simulink model "acc"  (R2021b)
settings: Solver=FixedStepAuto  StartTime=0.0  StopTime=206  FixedStep=0.0005  RelTol=1e-3
values from neighbouring files (symbols this model uses):
  Leftdis_PV_switch = 2    [acc_plot_backup.m]
  s_path = [0 1.10508939428 2.2141958029 3.32141571172 4.42705301151 5.53154548532 6.63517443471 7.73808041313 8.84055018688 9.94289959674 11.0453539299 12.1480581097 ... (1001 elements, 1001x1)]    [200_100radius.mat]    (also in LV_Clothoid_S_Turn_path.mat = [0 0.966832089581 1.93621320584 2.90214024471 3.86476766313 ; NEDC_path.mat = [0 0.414605943146 0.832514087334 1.25401518562 1.68216660344; Straight_East_into_curve.mat = [0 1.65770560069 3.32192925577 4.98420060507 6.64484613518 8; acc_plot_backup.m = Station_HV_m)
  X_path = [0 1.10508939428 2.2141958029 3.32141571172 4.42705301151 5.53154548532 6.63517443471 7.73808041313 8.84055018688 9.94289959674 11.0453539299 12.1480581097 ... (1001 elements, 1001x1)]    [200_100radius.mat]    (also in LV_Clothoid_S_Turn_path.mat = [-10 -9.03316791042 -8.06378679416 -7.09785975529 -6.1352323; NEDC_path.mat = [0 0.414605943146 0.832514087334 1.25401518562 1.68216660344; Straight_East_into_curve.mat = [0 1.65770560069 3.32192925577 4.98420060507 6.64484613518 8; acc_plot_backup.m = X_HV_m)
  Y_path = [0 -1.70364610795e-18 -7.41532896709e-18 1.46822109542e-17 4.74557362791e-17 6.12980216762e-17 9.25043977736e-17 1.24088240159e-16 1.5099156923e-16 1.7058517853e-16 1.90629227614e-16 2.09673434424e-16 ... (1001 elements, 1001x1)]    [200_100radius.mat]    (also in LV_Clothoid_S_Turn_path.mat = [0 -8.46153035536e-19 5.07382551045e-18 2.07356032218e-17 3.; NEDC_path.mat = [0 -3.50680326162e-18 -2.14111304971e-18 3.38197671014e-18 3; Straight_East_into_curve.mat = [0 1.29197709199e-18 2.81882429322e-18 3.49020462564e-17 6.7; acc_plot_backup.m = Y_HV_m)
undefined symbols (not defined in the file or in its folder): C_TICK_TIME_S, ENUM_ACCSTATE_DISABLED, ENUM_ACCSTATE_OFF, ENUM_ACCSTATE_STANDBY, FALSE, KVDI_ACCLongPressTime_ms, KVDI_ACCMaxActSpeed_kph, KVDI_ACCSetSpdIntial_kph, KVDI_ACCSpdLargeChange_kph, KVDI_LongPressConTime_ms, ONE_FLOAT, ONE_INT, R, Rw, T, TRUE, ZERO_FLOAT, ZERO_INT
libraries: simulink x16, dspstat3 x4, simulink_extras x2, Solver_SF x1
(part 2 of 4)

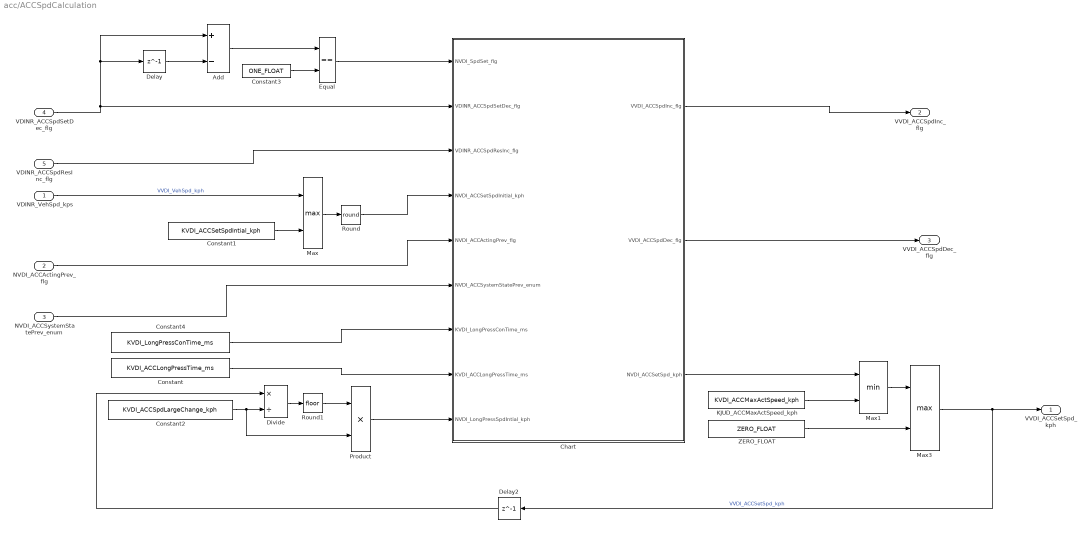
== system acc/ACCSpdCalculation ==
  VDINR_VehSpd_kps : Inport
  NVDI_ACCActingPrev_flg : Inport  Port=2
  NVDI_ACCSystemStatePrev_enum : Inport  Port=3
  VDINR_ACCSpdSetDec_flg : Inport  Port=4
  VDINR_ACCSpdResInc_flg : Inport  Port=5
  Add : Sum  Inputs=+-
  Chart : Stateflow chart  TreatAsAtomicUnit=on
      settings: PortSchema="{\"entries\":[{\"content\":{\"sides\":[{\"content\":{\"connectorIds\":[\"In1\",\"In2\",\"In3\",\"In4\",\"In5\",\"In6\",\"In9\",\"In7\",\"In8\"]},\"type\":\"ConnectorPlacement.EquallySpacedRectSide\",\"uuid\":\"b1b09059-7c6b-4f2a-a509-9d89abb69bff\"},{\"content\":{\"connectorIds\":[\"Out2\",\"Out3\",\"Out1\"],\"side\":\"RIGHT\"},\"type\":\"ConnectorPlacement.EquallySpacedRectSide\",\"uuid\":\"426eb2b7-8f84-437e-9ce1-b8172d5a5373\"},{\"content\":{\"connectorIds\":[],\"side\":\"TOP\"},\"type\":\"ConnectorPlacement.EquallySpacedRectSide\",\"uuid\":\"808310a0-6f78-4728-b2e8-69880cb1a9d0\"}]},\"type\":\"ConnectorPlacement.EquallySpacedConnector\",\"uuid\":\"50fcbb31-1c9a-4815-926e-b0772552613f\"}],\"packageUris\":[\"http://schema.mathworks.com/mf0/Connector/R2020b\"],\"version\":\"1.0\"}"
  Constant : Constant  Value=KVDI_ACCLongPressTime_ms
  Constant1 : Constant  Value=KVDI_ACCSetSpdIntial_kph
  Constant2 : Constant  Value=KVDI_ACCSpdLargeChange_kph
  Constant3 : Constant  Value=ONE_FLOAT
  Constant4 : Constant  Value=KVDI_LongPressConTime_ms
  Delay : Delay  DelayLength=1
  Delay2 : Delay  DelayLength=1
  Divide : Product  Inputs=*/
  Equal : RelationalOperator  Operator===  OutDataTypeStr=boolean  RndMeth=Simplest
  KJUD_ACCMaxActSpeed_kph : Constant  Value=KVDI_ACCMaxActSpeed_kph
  Max : MinMax  Function=max  Inputs=2
  Max1 : MinMax  Inputs=2
  Max3 : MinMax  Function=max  Inputs=2
  Product : Product
  Round : Rounding  Operator=round
  Round1 : Rounding
  ZERO_FLOAT : Constant  Value=ZERO_FLOAT
  VVDI_ACCSetSpd_kph : Outport
  VVDI_ACCSpdInc_flg : Outport  Port=2
  VVDI_ACCSpdDec_flg : Outport  Port=3
  wires:
  Constant4/1 -> Chart/9(KVDI_LongPressConTime_ms)
  Chart/2(VVDI_ACCSpdInc_flg) -> VVDI_ACCSpdInc_flg/1
  Chart/3(VVDI_ACCSpdDec_flg) -> VVDI_ACCSpdDec_flg/1
  Max1/1 -> Max3/1
  KJUD_ACCMaxActSpeed_kph/1 -> Max1/2
  VDINR_ACCSpdSetDec_flg/1 -> Chart/2(VDINR_ACCSpdSetDec_flg), Delay/1, Add/1
  Constant3/1 -> Equal/2
  Delay/1 -> Add/2
  Add/1 -> Equal/1
  Equal/1 -> Chart/1(NVDI_SpdSet_flg)
  ZERO_FLOAT/1 -> Max3/2
  Chart/1(NVDI_ACCSetSpd_kph) -> Max1/1
  Product/1 -> Chart/8(NVDI_LongPressSpdIntial_kph)
  Divide/1 -> Round1/1
  Round1/1 -> Product/1
  Constant2/1 -> Divide/2, Product/2
  Delay2/1 -> Divide/1
  Round/1 -> Chart/4(NVDI_ACCSetSpdInitial_kph)
  VDINR_VehSpd_kps/1 -> Max/1  "VVDI_VehSpd_kph"
  Constant1/1 -> Max/2
  Max/1 -> Round/1
  NVDI_ACCSystemStatePrev_enum/1 -> Chart/6(NVDI_ACCSystemStatePrev_enum)
  NVDI_ACCActingPrev_flg/1 -> Chart/5(NVDI_ACCActingPrev_flg)
  Max3/1 -> VVDI_ACCSetSpd_kph/1, Delay2/1  "VVDI_ACCSetSpd_kph"
  VDINR_ACCSpdResInc_flg/1 -> Chart/3(VDINR_ACCSpdResInc_flg)
  Constant/1 -> Chart/7(KVDI_ACCLongPressTime_ms)

== system acc/ACC_Mode_Selector ==
  ACCSetSpeed_mps : Inport
  VACCTargetVehNotAssigned_flg : Inport  Port=2
  RR : Inport  Port=3
  Vx_HV_mps : Inport  Port=4
  RV : Inport  Port=5
  Add : Sum
  Add13 : Sum  Inputs=+-
  Constant36 : Constant  Value=-0.5
  Logical Operator : Logic  Operator=OR  Inputs=3  AllPortsSameDT=off  OutDataTypeStr=boolean
  Logical Operator3 : Logic  AllPortsSameDT=off  OutDataTypeStr=boolean
  Relational Operator : RelationalOperator  Operator=<  OutDataTypeStr=boolean  RndMeth=Simplest
  Relational Operator1 : RelationalOperator  Operator=<  OutDataTypeStr=boolean  RndMeth=Simplest
  Relational Operator4 : RelationalOperator  Operator=<  OutDataTypeStr=boolean  RndMeth=Simplest
  TH_ref : Gain  Gain=1.5
  TH_ref4 : Gain  Gain=1.5
  dist_safe1 : Bias  Bias=-2
  Out1 : Outport
  wires:
  Logical Operator/1 -> Out1/1
  [Vx_PV_mps] -> Relational Operator/2
  VACCTargetVehNotAssigned_flg/1 -> Logical Operator/1
  Relational Operator/1 -> Logical Operator/2  "set_spd_compare"
  ACCSetSpeed_mps/1 -> [ACCSetSpeed_mps], Relational Operator/1
  Add/1 -> [Vx_PV_mps]
  Vx_HV_mps/1 -> [Vx_HV_mps], Add/2
  RV/1 -> Add/1
  dist_safe1/1 -> Add13/2, Relational Operator4/2  "act"
  TH_ref4/1 -> Relational Operator4/1  "des"
  Relational Operator1/1 -> Logical Operator3/1
  Constant36/1 -> Relational Operator1/2
  Add13/1 -> Relational Operator1/1
  Logical Operator3/1 -> Logical Operator/3  "dist_compare"
  RR/1 -> dist_safe1/1
  TH_ref/1 -> Add13/1  "des"
  [ACCSetSpeed_mps] -> TH_ref4/1
  [Vx_HV_mps] -> TH_ref/1
  Relational Operator4/1 -> Logical Operator3/2

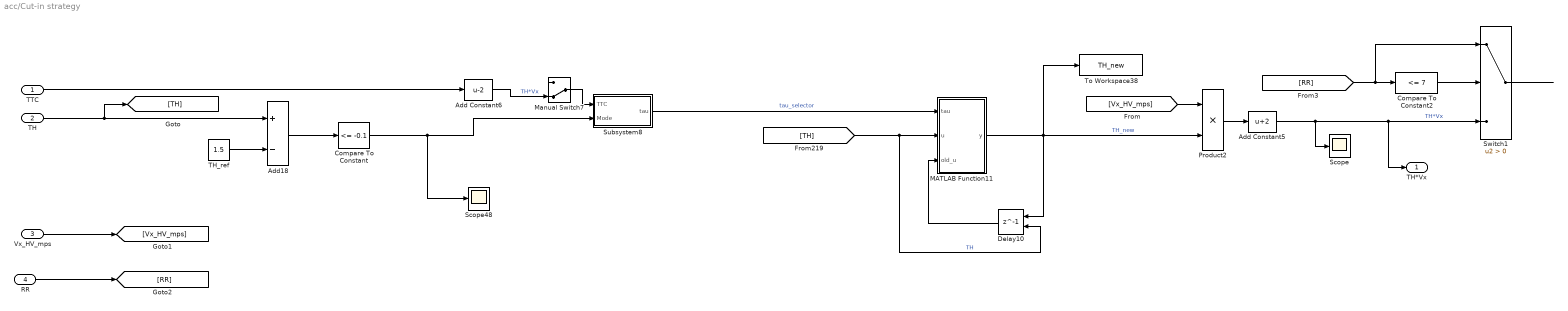
== system acc/Cut-in strategy ==
  TTC : Inport
  TH : Inport  Port=2
  Vx_HV_mps : Inport  Port=3
  RR : Inport  Port=4
  Add Constant5 : Bias  Bias=2
  Add Constant6 : Bias  Bias=-2
  Add18 : Sum  Inputs=+-
  Compare To Constant : simulink/Logic and Bit Operations/Compare To Constant  relop=<=  const=-0.1  OutDataTypeStr=boolean
  Compare To Constant2 : simulink/Logic and Bit Operations/Compare To Constant  relop=<=  const=7  OutDataTypeStr=boolean
  Delay10 : Delay  DelayLength=1  InitialConditionSource=Input port  SampleTime=0.1
      settings: InputPortMap=u0,p4
  MATLAB Function11 : MATLAB Function  TreatAsAtomicUnit=on
  Manual Switch7 : ManualSwitch  CurrentSetting=0
  Product2 : Product
  Scope : Scope
  Scope48 : Scope
  Subsystem8 : Subsystem
  Switch1 : Switch  Criteria=u2 > Threshold
  TH_ref : Constant  Value=1.5
  To Workspace38 : ToWorkspace  VariableName=TH_new  SampleTime=-1
  TH*Vx : Outport
  wires:
  [TH] -> Delay10/2, MATLAB Function11/2(u)  "TH"
  TH/1 -> Add18/1, [TH]
  Subsystem8/1(tau) -> MATLAB Function11/1(tau)  "tau_selector"
  Add18/1 -> Compare To Constant/1
  MATLAB Function11/1(y) -> Product2/2, To Workspace38/1, Delay10/1  "TH_new"
  Add Constant6/1 -> Manual Switch7/2  "TH*Vx"
  Delay10/1 -> MATLAB Function11/3(old_u)
  Product2/1 -> Add Constant5/1
  Manual Switch7/1 -> Subsystem8/1(TTC)
  TH_ref/1 -> Add18/2
  Compare To Constant/1 -> Scope48/1, Subsystem8/2(Mode)
  Add Constant5/1 -> Scope/1, TH*Vx/1, Switch1/3  "TH*Vx"
  [Vx_HV_mps] -> Product2/1
  TTC/1 -> Add Constant6/1
  Vx_HV_mps/1 -> [Vx_HV_mps]
  RR/1 -> [RR]
  [RR] -> Switch1/1, Compare To Constant2/1
  Compare To Constant2/1 -> Switch1/2
  Switch1/1 -> ?

== system acc/Latch ==
  set : Inport
  reset : Inport  Port=2
  Delay : Delay  DelayLength=1
  Logical Operator3 : Logic  AllPortsSameDT=off  OutDataTypeStr=boolean
  Logical Operator4 : Logic  Operator=NOT  AllPortsSameDT=off  OutDataTypeStr=boolean
  Switch : Switch  Criteria=u2 ~= 0
  Switch1 : Switch  Criteria=u2 ~= 0
  latched : Outport
  wires:
  Delay/1 -> Switch1/3
  Logical Operator4/1 -> Logical Operator3/2, Switch1/1
  Logical Operator3/1 -> Switch/2
  reset/1 -> Logical Operator4/1, Switch1/2
  Switch/1 -> Delay/1, latched/1
  set/1 -> Switch/1, Logical Operator3/1
  Switch1/1 -> Switch/3

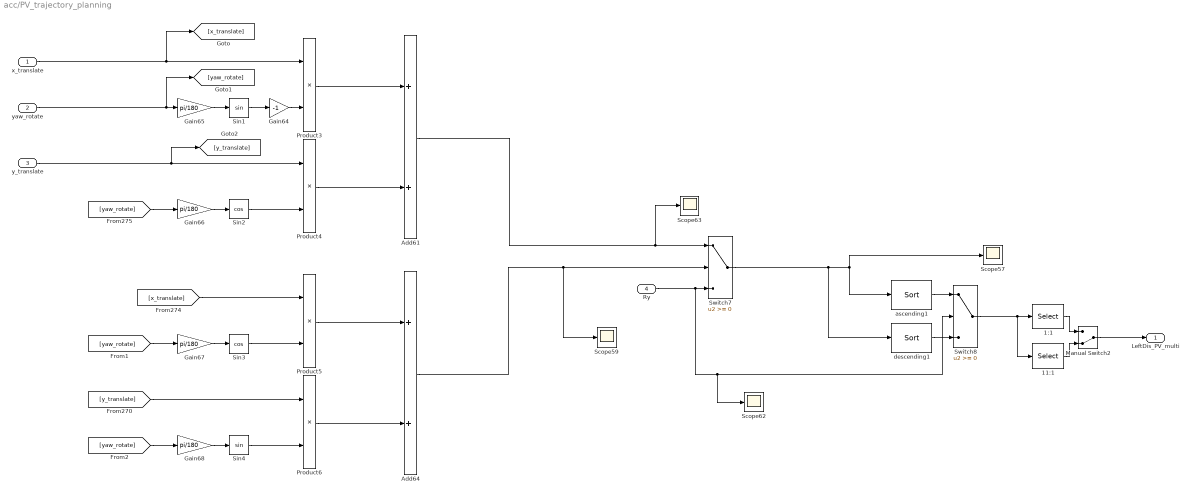
== system acc/PV_trajectory_planning ==
  x_translate : Inport
  yaw_rotate : Inport  Port=2
  y_translate : Inport  Port=3
  Ry : Inport  Port=4
  11:1 : Selector  InputPortWidth=20  IndexOptions=Index vector (dialog)  Indices=[11:20]  OutputSizes=1
  1:1 : Selector  InputPortWidth=20  IndexOptions=Index vector (dialog)  Indices=[1:10]  OutputSizes=1
  Add61 : Sum
  Add64 : Sum
  Gain64 : Gain  Gain=-1
  Gain{65..68} (4 alike) : Gain  Gain=pi/180
  Manual Switch2 : ManualSwitch  CurrentSetting=0
  Product{3..6} (4 alike) : Product
  Scope{57,59,62..63} (4 alike) : Scope
  Sin1 : Trigonometry
  Sin2 : Trigonometry  Operator=cos
  Sin3 : Trigonometry  Operator=cos
  Sin4 : Trigonometry
  Switch7 : Switch
  Switch8 : Switch
  ascending1 : dspstat3/Sort  otype=Value  dir=Ascending  sortAlg=Quick sort  roundingMode=Floor  overflowMode=off  accumDataTypeStr=Inherit: Same as product output  accumLastDataTypeStr=Inherit: Same as product output
      settings: SourceProductBaseCode=DS
  descending1 : dspstat3/Sort  otype=Value  dir=Descending  sortAlg=Quick sort  roundingMode=Floor  overflowMode=off  accumDataTypeStr=Inherit: Same as product output  accumLastDataTypeStr=Inherit: Same as product output
      settings: SourceProductBaseCode=DS
  LeftDis_PV_multi : Outport
  wires:
  Add64/1 -> Scope59/1, Switch7/2
  Product5/1 -> Add64/1
  Gain68/1 -> Sin4/1
  Sin1/1 -> Gain64/1
  Gain64/1 -> Product3/2
  descending1/1 -> Switch8/3
  Ry/1 -> Scope62/1, Switch8/2, Switch7/3
  Sin4/1 -> Product6/2
  Gain67/1 -> Sin3/1
  Switch8/1 -> 11:1/1, 1:1/1
  [yaw_rotate] -> Gain68/1
  Sin3/1 -> Product5/2
  Product6/1 -> Add64/2
  Switch7/1 -> Scope57/1, ascending1/1, descending1/1
  Sin2/1 -> Product4/2
  Gain66/1 -> Sin2/1
  y_translate/1 -> [y_translate], Product4/1
  Gain65/1 -> Sin1/1
  [x_translate] -> Product5/1
  ascending1/1 -> Switch8/1
  1:1/1 -> Manual Switch2/1
  Product4/1 -> Add61/2
  11:1/1 -> Manual Switch2/2
  Add61/1 -> Scope63/1, Switch7/1
  Product3/1 -> Add61/1
  Manual Switch2/1 -> LeftDis_PV_multi/1
  x_translate/1 -> Product3/1, [x_translate]
  [y_translate] -> Product6/1
  [yaw_rotate] -> Gain67/1
  yaw_rotate/1 -> [yaw_rotate], Gain65/1
  [yaw_rotate] -> Gain66/1

== system acc/R selector ==
  In1 : Inport
  vx : Inport  Port=2
  1-D Lookup Table2 : Lookup_n-D  NumberOfTableDimensions=1  BreakpointsForDimension1=[0 15 28 40]/3.6  Table=[31 31 35 35]  InternalRulePriority=Speed  RndMeth=Simplest  InputSameDT=on
  Constant1 : Constant  Value=35
  Constant19 : Constant
  Constant2 : Constant  Value=20
  Constant66 : Constant  Value=0.5
  Switch12 : Switch  Criteria=u2 > Threshold
  Out1 : Outport
  wires:
  Constant66/1 -> Switch12/1
  1-D Lookup Table2/1 -> Switch12/3
  In1/1 -> Switch12/2
  Switch12/1 -> Out1/1
  vx/1 -> 1-D Lookup Table2/1

== system acc/R selector1 ==
  In1 : Inport
  vx : Inport  Port=2
  1-D Lookup Table2 : Lookup_n-D  NumberOfTableDimensions=1  BreakpointsForDimension1=[0 15 28 40]/3.6  Table=[31 31 35 35]  InternalRulePriority=Speed  RndMeth=Simplest  InputSameDT=on
  Constant1 : Constant  Value=35
  Constant19 : Constant
  Constant2 : Constant  Value=7
  Constant66 : Constant  Value=0.5
  Switch12 : Switch  Criteria=u2 > Threshold
  Out1 : Outport
  wires:
  Switch12/1 -> Out1/1
  In1/1 -> Switch12/2
  Constant2/1 -> Switch12/3
  Constant66/1 -> Switch12/1

== system acc/Smooth Switch ==
  Spd_acc_cmd : Inport
  Mode : Inport  Port=2
  TH_acc_cmd : Inport  Port=3
  TTC : Inport  Port=4
  Add12 : Sum
  Add9 : Sum  Inputs=+-
  Constant49 : Constant
  Data Type Conversion : DataTypeConversion  OutDataTypeStr=double
  Delay : Delay  DelayLength=1  InitialConditionSource=Input port  SampleTime=0.1
      settings: InputPortMap=u0,p4
  MATLAB Function : MATLAB Function  TreatAsAtomicUnit=on
  Product1 : Product
  Product2 : Product
  Scope : Scope
  Subsystem : Subsystem
  ax_cmd : Outport
  wires:
  Product2/1 -> Add12/1
  Spd_acc_cmd/1 -> Product2/1
  MATLAB Function/1(y) -> Delay/1, Scope/1, Add9/2, Product2/2
  Data Type Conversion/1 -> Delay/2, MATLAB Function/2(u)
  Constant49/1 -> Add9/1
  Product1/1 -> Add12/2
  TH_acc_cmd/1 -> Product1/2
  Add9/1 -> Product1/1
  Add12/1 -> ax_cmd/1
  Mode/1 -> Subsystem/2(Mode), Data Type Conversion/1
  Delay/1 -> MATLAB Function/3(old_u)
  Subsystem/1(tau) -> MATLAB Function/1(tau)  "tau_selector"
  TTC/1 -> Subsystem/1(TTC)

== system acc/Smooth Switch1 ==
  Dynamic_cmd : Inport
  Mode : Inport  Port=2
  Kinematic_cmd : Inport  Port=3
  Add12 : Sum
  Add9 : Sum  Inputs=+-
  Constant49 : Constant
  Data Type Conversion : DataTypeConversion  OutDataTypeStr=double
  Product1 : Product
  Product2 : Product
  Transfer Fcn5 : TransferFcn  Denominator=[0.5 1]
  ax_cmd : Outport
  wires:
  Mode/1 -> Data Type Conversion/1
  Add12/1 -> ax_cmd/1
  Add9/1 -> Product1/1
  Kinematic_cmd/1 -> Product1/2
  Product1/1 -> Add12/2
  Constant49/1 -> Add9/1
  Data Type Conversion/1 -> Transfer Fcn5/1
  Transfer Fcn5/1 -> Product2/2, Add9/2
  Dynamic_cmd/1 -> Product2/1
  Product2/1 -> Add12/1

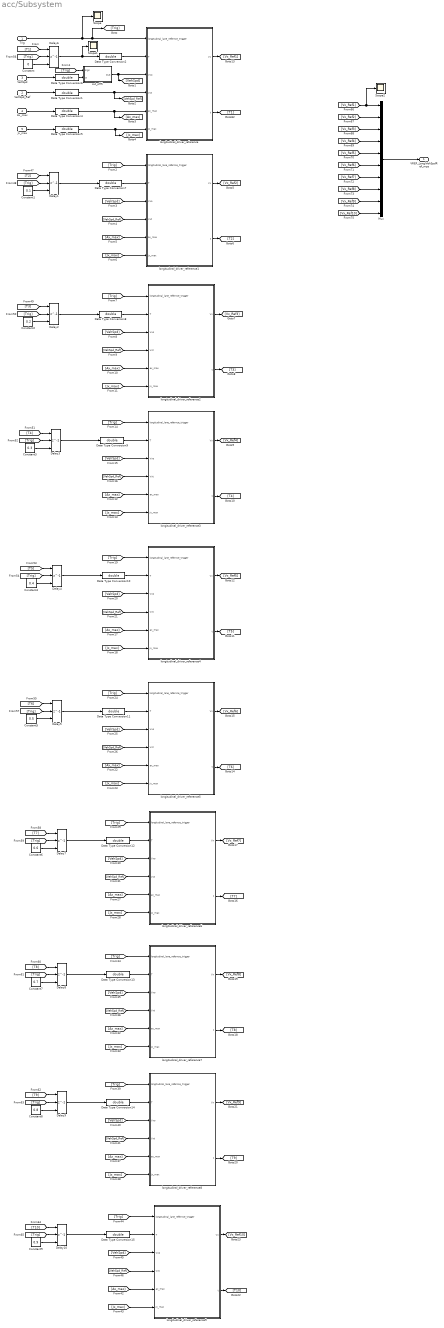
== system acc/Subsystem ==
  "Trig " : Inport
  VehSpd_Ref : Inport  Port=2
  VehSpd : Inport  Port=3
  Ax_max : Inport  Port=4
  Jx_max : Inport  Port=5
  Constant : Constant  Value=0
  Constant1 : Constant  Value=0.1
  Constant2 : Constant  Value=0.2
  Constant3 : Constant  Value=0.3
  Constant4 : Constant  Value=0.4
  Constant5 : Constant  Value=0.5
  Constant6 : Constant  Value=0.6
  Constant7 : Constant  Value=0.7
  Constant8 : Constant  Value=0.8
  Constant9 : Constant  Value=0.9
  Data Type Conversion{1..2,4..15} (14 alike) : DataTypeConversion  OutDataTypeStr=double
  Delay{1..10} (10 alike) : Delay  DelayLength=1  InitialConditionSource=Input port  ExternalReset=Rising
      settings: InputPortMap=u0,r5,p4
  Mux : Mux  Inputs=10
  Scope : Scope
  Scope1 : Scope
  Scope2 : Scope
  cut_off5 : Subsystem
  longitudinal_driver_reference : MATLAB Function  TreatAsAtomicUnit=on
  longitudinal_driver_reference1 : MATLAB Function  TreatAsAtomicUnit=on
  longitudinal_driver_reference2 : MATLAB Function  TreatAsAtomicUnit=on
  longitudinal_driver_reference3 : MATLAB Function  TreatAsAtomicUnit=on
  longitudinal_driver_reference4 : MATLAB Function  TreatAsAtomicUnit=on
  longitudinal_driver_reference5 : MATLAB Function  TreatAsAtomicUnit=on
  longitudinal_driver_reference6 : MATLAB Function  TreatAsAtomicUnit=on
  longitudinal_driver_reference7 : MATLAB Function  TreatAsAtomicUnit=on
  longitudinal_driver_reference8 : MATLAB Function  TreatAsAtomicUnit=on
  longitudinal_driver_reference9 : MATLAB Function  TreatAsAtomicUnit=on
  "VREF_LongiVehSpdRef_mps " : Outport
  wires:
  longitudinal_driver_reference/1(Vx) -> [Vx_Ref1]
  Mux/1 -> "VREF_LongiVehSpdRef_mps "/1
  Constant/1 -> Delay6/3
  [T1] -> Delay6/1
  Ax_max/1 -> Data Type Conversion4/1
  Jx_max/1 -> Data Type Conversion5/1
  VehSpd_Ref/1 -> Data Type Conversion1/1
  longitudinal_driver_reference/2(t) -> [T1]
  Delay6/1 -> Scope1/1, Data Type Conversion2/1
  [Trig] -> Delay6/2
  "Trig "/1 -> Scope/1, [Trig], longitudinal_driver_reference/1(longitudinal_lane_refernce_trigger)
  Data Type Conversion2/1 -> longitudinal_driver_reference/2(T)
  VehSpd/1 -> Data Type Conversion6/1
  Data Type Conversion1/1 -> [VehSpd_Ref], longitudinal_driver_reference/4(Vxt)
  cut_off5/1(Out) -> [VehSpd], longitudinal_driver_reference/3(Vxo)
  Data Type Conversion6/1 -> cut_off5/2(in)
  [Trig] -> cut_off5/1(sign)
  Data Type Conversion5/1 -> [Jx_max], longitudinal_driver_reference/6(jx_max)
  Data Type Conversion4/1 -> [Ax_max], longitudinal_driver_reference/5(ax_max)
  [Trig] -> longitudinal_driver_reference1/1(longitudinal_lane_refernce_trigger)
  [VehSpd] -> longitudinal_driver_reference1/3(Vxo)
  [VehSpd_Ref] -> longitudinal_driver_reference1/4(Vxt)
  [Ax_max] -> longitudinal_driver_reference1/5(ax_max)
  [Jx_max] -> longitudinal_driver_reference1/6(jx_max)
  [Jx_max] -> longitudinal_driver_reference2/6(jx_max)
  [Ax_max] -> longitudinal_driver_reference2/5(ax_max)
  [VehSpd_Ref] -> longitudinal_driver_reference2/4(Vxt)
  [VehSpd] -> longitudinal_driver_reference2/3(Vxo)
  [Trig] -> longitudinal_driver_reference2/1(longitudinal_lane_refernce_trigger)
  [Trig] -> longitudinal_driver_reference3/1(longitudinal_lane_refernce_trigger)
  [VehSpd] -> longitudinal_driver_reference3/3(Vxo)
  [VehSpd_Ref] -> longitudinal_driver_reference3/4(Vxt)
  [Ax_max] -> longitudinal_driver_reference3/5(ax_max)
  [Jx_max] -> longitudinal_driver_reference3/6(jx_max)
  [Jx_max] -> longitudinal_driver_reference4/6(jx_max)
  [Ax_max] -> longitudinal_driver_reference4/5(ax_max)
  [VehSpd_Ref] -> longitudinal_driver_reference4/4(Vxt)
  [VehSpd] -> longitudinal_driver_reference4/3(Vxo)
  [Trig] -> longitudinal_driver_reference4/1(longitudinal_lane_refernce_trigger)
  [Trig] -> longitudinal_driver_reference5/1(longitudinal_lane_refernce_trigger)
  [VehSpd] -> longitudinal_driver_reference5/3(Vxo)
  [VehSpd_Ref] -> longitudinal_driver_reference5/4(Vxt)
  [Ax_max] -> longitudinal_driver_reference5/5(ax_max)
  [Jx_max] -> longitudinal_driver_reference5/6(jx_max)
  [Jx_max] -> longitudinal_driver_reference6/6(jx_max)
  [Ax_max] -> longitudinal_driver_reference6/5(ax_max)
  [VehSpd_Ref] -> longitudinal_driver_reference6/4(Vxt)
  [VehSpd] -> longitudinal_driver_reference6/3(Vxo)
  [Trig] -> longitudinal_driver_reference6/1(longitudinal_lane_refernce_trigger)
  [Trig] -> longitudinal_driver_reference7/1(longitudinal_lane_refernce_trigger)
  [VehSpd] -> longitudinal_driver_reference7/3(Vxo)
  [VehSpd_Ref] -> longitudinal_driver_reference7/4(Vxt)
  [Ax_max] -> longitudinal_driver_reference7/5(ax_max)
  [Jx_max] -> longitudinal_driver_reference7/6(jx_max)
  [Jx_max] -> longitudinal_driver_reference8/6(jx_max)
  [Ax_max] -> longitudinal_driver_reference8/5(ax_max)
  [VehSpd_Ref] -> longitudinal_driver_reference8/4(Vxt)
  [VehSpd] -> longitudinal_driver_reference8/3(Vxo)
  [Trig] -> longitudinal_driver_reference8/1(longitudinal_lane_refernce_trigger)
  [Trig] -> longitudinal_driver_reference9/1(longitudinal_lane_refernce_trigger)
  [VehSpd] -> longitudinal_driver_reference9/3(Vxo)
  [VehSpd_Ref] -> longitudinal_driver_reference9/4(Vxt)
  [Ax_max] -> longitudinal_driver_reference9/5(ax_max)
  [Jx_max] -> longitudinal_driver_reference9/6(jx_max)
  longitudinal_driver_reference1/1(Vx) -> [Vx_Ref2]
  longitudinal_driver_reference1/2(t) -> [T2]
  [Trig] -> Delay1/2
  Delay1/1 -> Data Type Conversion7/1
  [T2] -> Delay1/1
  Data Type Conversion7/1 -> longitudinal_driver_reference1/2(T)
  Constant1/1 -> Delay1/3
  Constant2/1 -> Delay2/3
  Data Type Conversion8/1 -> longitudinal_driver_reference2/2(T)
  [T3] -> Delay2/1
  Delay2/1 -> Data Type Conversion8/1
  [Trig] -> Delay2/2
  longitudinal_driver_reference2/2(t) -> [T3]
  longitudinal_driver_reference2/1(Vx) -> [Vx_Ref3]
  [Trig] -> Delay3/2
  Delay3/1 -> Data Type Conversion9/1
  [T4] -> Delay3/1
  Data Type Conversion9/1 -> longitudinal_driver_reference3/2(T)
  Constant3/1 -> Delay3/3
  longitudinal_driver_reference3/1(Vx) -> [Vx_Ref4]
  longitudinal_driver_reference3/2(t) -> [T4]
  Constant4/1 -> Delay4/3
  Data Type Conversion10/1 -> longitudinal_driver_reference4/2(T)
  [T5] -> Delay4/1
  Delay4/1 -> Data Type Conversion10/1
  [Trig] -> Delay4/2
  longitudinal_driver_reference4/2(t) -> [T5]
  longitudinal_driver_reference4/1(Vx) -> [Vx_Ref5]
  longitudinal_driver_reference5/1(Vx) -> [Vx_Ref6]
  longitudinal_driver_reference5/2(t) -> [T6]
  [Trig] -> Delay5/2
  Delay5/1 -> Data Type Conversion11/1
  [T6] -> Delay5/1
  Constant5/1 -> Delay5/3
  Data Type Conversion11/1 -> longitudinal_driver_reference5/2(T)
  longitudinal_driver_reference6/2(t) -> [T7]
  longitudinal_driver_reference6/1(Vx) -> [Vx_Ref7]
  Constant6/1 -> Delay7/3
  [T7] -> Delay7/1
  Delay7/1 -> Data Type Conversion12/1
  [Trig] -> Delay7/2
  Data Type Conversion12/1 -> longitudinal_driver_reference6/2(T)
  [Trig] -> Delay8/2
  Delay8/1 -> Data Type Conversion13/1
  [T8] -> Delay8/1
  Constant7/1 -> Delay8/3
  Data Type Conversion13/1 -> longitudinal_driver_reference7/2(T)
  longitudinal_driver_reference7/1(Vx) -> [Vx_Ref8]
  longitudinal_driver_reference7/2(t) -> [T8]
  longitudinal_driver_reference8/2(t) -> [T9]
  longitudinal_driver_reference8/1(Vx) -> [Vx_Ref9]
  Data Type Conversion14/1 -> longitudinal_driver_reference8/2(T)
  Constant8/1 -> Delay9/3
  [T9] -> Delay9/1
  Delay9/1 -> Data Type Conversion14/1
  [Trig] -> Delay9/2
  longitudinal_driver_reference9/1(Vx) -> [Vx_Ref10]
  longitudinal_driver_reference9/2(t) -> [T10]
  [Trig] -> Delay10/2
  Delay10/1 -> Data Type Conversion15/1
  [T10] -> Delay10/1
  Constant9/1 -> Delay10/3
  Data Type Conversion15/1 -> longitudinal_driver_reference9/2(T)
  [Vx_Ref1] -> Scope2/1, Mux/1
  [Vx_Ref2] -> Mux/2
  [Vx_Ref3] -> Mux/3
  [Vx_Ref4] -> Mux/4
  [Vx_Ref5] -> Mux/5
  [Vx_Ref6] -> Mux/6
  [Vx_Ref7] -> Mux/7
  [Vx_Ref8] -> Mux/8
  [Vx_Ref9] -> Mux/9
  [Vx_Ref10] -> Mux/10

== system acc/Subsystem1 ==
  In1 : Inport
  Constant117 : Constant  Value=single(1)  OutDataTypeStr=single
  Relational Operator : RelationalOperator  OutDataTypeStr=boolean  RndMeth=Simplest
  Saturation5 : Saturate  UpperLimit=inf  LowerLimit=40/3.6
  Switch7 : Switch  Criteria=u2 ~= 0
  Out1 : Outport
  wires:
  Relational Operator/1 -> Switch7/2
  In1/1 -> Relational Operator/1, Switch7/1
  Constant117/1 -> Relational Operator/2, Switch7/3
  Switch7/1 -> Out1/1

== system acc/Subsystem16 ==
  C0 : Inport
  C1 : Inport  Port=2
  "C2 " : Inport  Port=3
  C3 : Inport  Port=4
  PrediDis : Inport  Port=5
  Add30 : Sum  Inputs=++++
  Fcn : Fcn  Expr=(u)^3
  Product : Product
  Product1 : Product
  Product2 : Product
  Square : Math  Operator=square  SignedPower=on  RndMeth=Zero  SaturateOnIntegerOverflow=on
  LeftDis : Outport  VectorParamsAs1DForOutWhenUnconnected=off
  wires:
  PrediDis/1 -> [PrediDis]
  [PrediDis] -> Square/1
  Product/1 -> Add30/2
  Product1/1 -> Add30/3
  "C2 "/1 -> Product1/1
  [PrediDis] -> Product/2
  [PrediDis] -> Fcn/1
  Fcn/1 -> Product2/2
  Square/1 -> Product1/2
  C0/1 -> Add30/1
  Product2/1 -> Add30/4
  C1/1 -> Product/1
  Add30/1 -> LeftDis/1
  C3/1 -> Product2/1

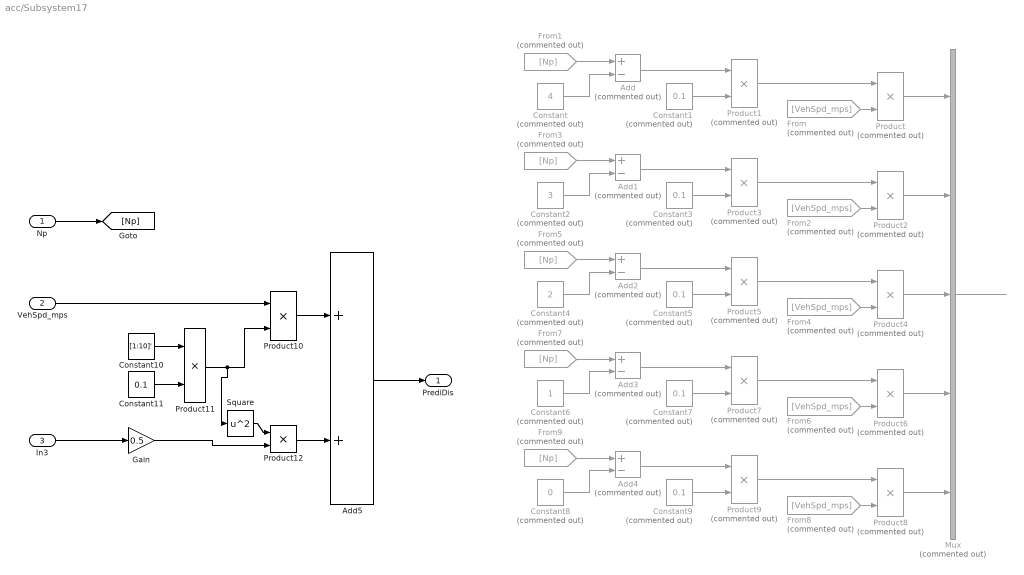
== system acc/Subsystem17 ==
  Np : Inport
  VehSpd_mps : Inport  Port=2
  In3 : Inport  Port=3
  Add{,1..4} (5 alike) : Sum  Commented=on  Inputs=+-
  Add5 : Sum
  Constant : Constant  Commented=on  Value=4
  Constant{1,3,5,7,9} (5 alike) : Constant  Commented=on  Value=0.1
  Constant10 : Constant  Value=[1:10]'
  Constant11 : Constant  Value=0.1
  Constant2 : Constant  Commented=on  Value=3
  Constant4 : Constant  Commented=on  Value=2
  Constant6 : Constant  Commented=on
  Constant8 : Constant  Commented=on  Value=0
  From{,2,4,6,8} (5 alike) : From  Commented=on  GotoTag=VehSpd_mps
  From{1,3,5,7,9} (5 alike) : From  Commented=on  GotoTag=Np
  Gain : Gain  Gain=0.5
  Mux : Mux  Commented=on  Inputs=5
  Product{,1..9} (10 alike) : Product  Commented=on
  Product10 : Product
  Product11 : Product
  Product12 : Product
  Square : Math  Operator=square  SaturateOnIntegerOverflow=on
  PrediDis : Outport  VectorParamsAs1DForOutWhenUnconnected=off
  wires:
  Product8/1 -> Mux/5
  Constant9/1 -> Product9/2
  Constant8/1 -> Add4/2
  From9/1 -> Add4/1
  Add4/1 -> Product9/1
  Product9/1 -> Product8/1
  From8/1 -> Product8/2
  From6/1 -> Product6/2
  Product7/1 -> Product6/1
  Add3/1 -> Product7/1
  From7/1 -> Add3/1
  Constant6/1 -> Add3/2
  Constant7/1 -> Product7/2
  Product6/1 -> Mux/4
  Product4/1 -> Mux/3
  Constant5/1 -> Product5/2
  Constant4/1 -> Add2/2
  From5/1 -> Add2/1
  Add2/1 -> Product5/1
  Product5/1 -> Product4/1
  From4/1 -> Product4/2
  Product2/1 -> Mux/2
  From2/1 -> Product2/2
  Product3/1 -> Product2/1
  Add1/1 -> Product3/1
  From3/1 -> Add1/1
  Constant2/1 -> Add1/2
  Constant3/1 -> Product3/2
  Constant1/1 -> Product1/2
  Constant/1 -> Add/2
  From1/1 -> Add/1
  Add/1 -> Product1/1
  Product1/1 -> Product/1
  From/1 -> Product/2
  Product/1 -> Mux/1
  Np/1 -> [Np]
  Mux/1 -> ?
  Product10/1 -> Add5/1
  VehSpd_mps/1 -> Product10/1
  Product11/1 -> Product10/2, Square/1
  Constant10/1 -> Product11/1
  Constant11/1 -> Product11/2
  Add5/1 -> PrediDis/1
  In3/1 -> Gain/1
  Product12/1 -> Add5/2
  Square/1 -> Product12/1
  Gain/1 -> Product12/2

== system acc/Subsystem2 ==
  T_cmd : Inport
  Gain : Gain  Gain=-0.25
  Gain2 : Gain  Gain=1/250
  Gain3 : Gain  Gain=1/150
  Saturation1 : Saturate  UpperLimit=0  LowerLimit=-inf
  Smooth_Switch1 : Subsystem  Commented=on  mask{tau=0.3, IC=0, T=0.1}
      mask prompts: tau "Time constant"; T "Sample time"
      mask Display:
      | fprintf('Discrete first order \n\n')
      | fprintf(['tau=' num2str(tau) '    IC=' num2str(IC)])
  Transfer Fcn1 : TransferFcn  Denominator=[0.3 1]
  Transfer Fcn2 : TransferFcn  Denominator=[0.3 1]
  Pb_LF : Outport
  Pb_RF : Outport  Port=2
  Pb_RL : Outport  Port=3
  Pb_RR : Outport  Port=4
  wires:
  Transfer Fcn1/1 -> Pb_RR/1, Pb_RL/1
  Transfer Fcn2/1 -> Pb_RF/1, Pb_LF/1
  Gain3/1 -> Transfer Fcn1/1
  Gain2/1 -> Transfer Fcn2/1
  Gain/1 -> Gain2/1, Gain3/1
  Saturation1/1 -> Gain/1
  T_cmd/1 -> Saturation1/1

== system acc/Subsystem3 ==
  Jerk : Inport
  Vx : Inport  Port=2
  Constant1 : Constant  Value=0  OutDataTypeStr=single
  Constant117 : Constant  Value=0.5  OutDataTypeStr=single
  Relational Operator : RelationalOperator  OutDataTypeStr=boolean  RndMeth=Simplest
  Switch7 : Switch  Criteria=u2 ~= 0
  Out1 : Outport
  wires:
  Relational Operator/1 -> Switch7/2
  Vx/1 -> Relational Operator/1
  Constant117/1 -> Relational Operator/2
  Switch7/1 -> Out1/1
  Constant1/1 -> Switch7/3
  Jerk/1 -> Switch7/1

== system acc/Subsystem4 ==
  new_value : Inport
  Constant44 : Constant  Value=0.25
  Constant48 : Constant  Value=0.1
  Delay1 : Delay  DelayLength=1  SampleTime=0.1
  rolling_avg1 : Subsystem
  new_ave : Outport
  wires:
  Constant44/1 -> rolling_avg1/4(tc)
  new_value/1 -> rolling_avg1/1(new_value)
  Constant48/1 -> rolling_avg1/3(delta_t)  "T"
  Delay1/1 -> rolling_avg1/2(old_ave)
  rolling_avg1/1(new_ave) -> new_ave/1, Delay1/1

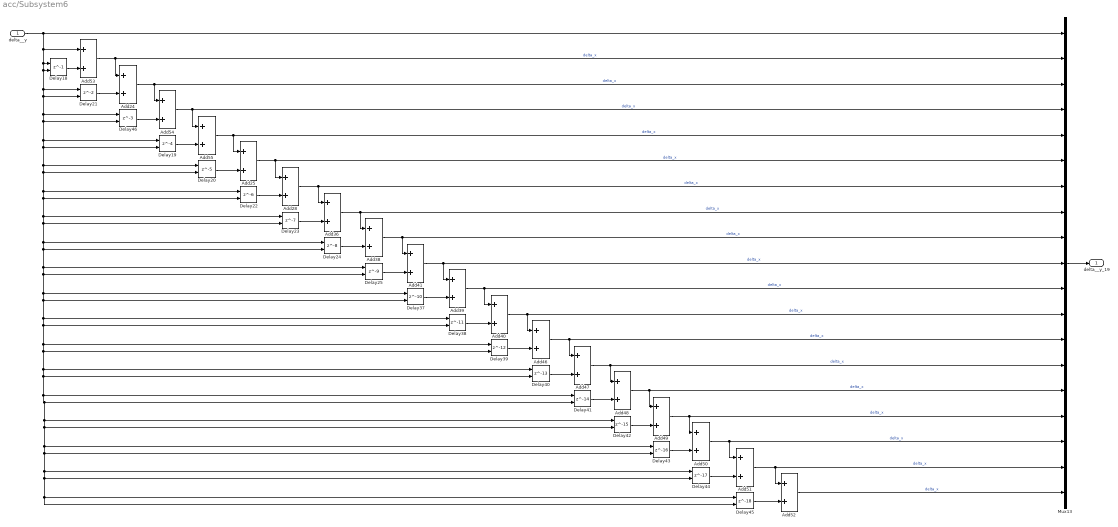
== system acc/Subsystem6 ==
  delta__y : Inport
  Add{24..25,28,36,38..41,46..55} (18 alike) : Sum
  Delay18 : Delay  DelayLength=1  InitialConditionSource=Input port
      settings: InputPortMap=u0,p4
  Delay19 : Delay  DelayLength=4  InitialConditionSource=Input port
      settings: InputPortMap=u0,p4
  Delay20 : Delay  DelayLength=5  InitialConditionSource=Input port
      settings: InputPortMap=u0,p4
  Delay21 : Delay  InitialConditionSource=Input port
      settings: InputPortMap=u0,p4
  Delay22 : Delay  DelayLength=6  InitialConditionSource=Input port
      settings: InputPortMap=u0,p4
  Delay23 : Delay  DelayLength=7  InitialConditionSource=Input port
      settings: InputPortMap=u0,p4
  Delay24 : Delay  DelayLength=8  InitialConditionSource=Input port
      settings: InputPortMap=u0,p4
  Delay25 : Delay  DelayLength=9  InitialConditionSource=Input port
      settings: InputPortMap=u0,p4
  Delay37 : Delay  DelayLength=10  InitialConditionSource=Input port
      settings: InputPortMap=u0,p4
  Delay38 : Delay  DelayLength=11  InitialConditionSource=Input port
      settings: InputPortMap=u0,p4
  Delay39 : Delay  DelayLength=12  InitialConditionSource=Input port
      settings: InputPortMap=u0,p4
  Delay40 : Delay  DelayLength=13  InitialConditionSource=Input port
      settings: InputPortMap=u0,p4
  Delay41 : Delay  DelayLength=14  InitialConditionSource=Input port
      settings: InputPortMap=u0,p4
  Delay42 : Delay  DelayLength=15  InitialConditionSource=Input port
      settings: InputPortMap=u0,p4
  Delay43 : Delay  DelayLength=16  InitialConditionSource=Input port
      settings: InputPortMap=u0,p4
  Delay44 : Delay  DelayLength=17  InitialConditionSource=Input port
      settings: InputPortMap=u0,p4
  Delay45 : Delay  DelayLength=18  InitialConditionSource=Input port
      settings: InputPortMap=u0,p4
  Delay46 : Delay  DelayLength=3  InitialConditionSource=Input port
      settings: InputPortMap=u0,p4
  Mux13 : Mux  Inputs=19
  delta__y_19 : Outport
  wires:
  Delay21/1 -> Add24/2
  delta__y/1 -> Mux13/1, Delay21/2, Delay46/1, Delay22/1, Delay25/2, Delay37/1, Delay39/2, Delay40/1, Delay41/1, Delay42/1, Delay42/2, Delay43/1, Delay44/1, Delay45/1, Delay45/2, Delay44/2, Delay43/2, Delay41/2, Delay40/2, Delay39/1, Delay38/2, Delay38/1, Delay37/2, Delay25/1, Delay24/2, Delay24/1, Delay23/2, Delay23/1, Delay22/2, Delay20/2, Delay20/1, Delay19/2, Delay19/1, Delay46/2, Delay21/1, Delay18/2, Delay18/1, Add53/1
  Delay22/1 -> Add28/2
  Add46/1 -> Mux13/13, Add47/1  "delta_x"
  Delay37/1 -> Add39/2
  Add39/1 -> Mux13/11, Add40/1  "delta_x"
  Delay38/1 -> Add40/2
  Add40/1 -> Mux13/12, Add46/1  "delta_x"
  Add38/1 -> Mux13/9, Add41/1  "delta_x"
  Add53/1 -> Mux13/2, Add24/1  "delta_x"
  Add55/1 -> Mux13/5, Add25/1  "delta_x"
  Add50/1 -> Add51/1, Mux13/17  "delta_x"
  Add47/1 -> Mux13/14, Add48/1  "delta_x"
  Delay39/1 -> Add46/2
  Delay40/1 -> Add47/2
  Mux13/1 -> delta__y_19/1
  Delay46/1 -> Add54/2
  Delay25/1 -> Add41/2
  Add52/1 -> Mux13/19  "delta_x"
  Add28/1 -> Mux13/7, Add36/1  "delta_x"
  Add36/1 -> Mux13/8, Add38/1  "delta_x"
  Delay23/1 -> Add36/2
  Delay20/1 -> Add25/2
  Delay42/1 -> Add49/2
  Delay44/1 -> Add51/2
  Delay18/1 -> Add53/2
  Add25/1 -> Mux13/6, Add28/1  "delta_x"
  Add41/1 -> Mux13/10, Add39/1  "delta_x"
  Add49/1 -> Add50/1, Mux13/16  "delta_x"
  Add51/1 -> Add52/1, Mux13/18  "delta_x"
  Delay19/1 -> Add55/2
  Add24/1 -> Mux13/3, Add54/1  "delta_x"
  Delay45/1 -> Add52/2
  Delay41/1 -> Add48/2
  Add54/1 -> Mux13/4, Add55/1  "delta_x"
  Delay24/1 -> Add38/2
  Delay43/1 -> Add50/2
  Add48/1 -> Mux13/15, Add49/1  "delta_x"

== system acc/V_rel Estimation ==
  cut_in_flg : Inport
  a_c : Inport  Port=2
  S_rel : Inport  Port=3
  initial_value : Inport  Port=4
  Add3 : Sum  Inputs=-+
  Delay1 : Delay  DelayLength=1  InitialConditionSource=Input port  SampleTime=0.1
      settings: InputPortMap=u0,p4
  Kalman filter : Subsystem
  sample time : Gain  Gain=1/0.1
  s_rel : Outport
  v_rel : Outport  Port=2
  a_rel : Outport  Port=3
  wires:
  S_rel/1 -> Kalman filter/3(S_rel)
  Kalman filter/1(s_rel) -> s_rel/1
  Add3/1 -> sample time/1
  Delay1/1 -> Add3/1
  a_c/1 -> Delay1/1, Delay1/2, Add3/2
  Kalman filter/2(v_rel) -> v_rel/1
  sample time/1 -> Kalman filter/2(Jerk)  "Jerk"
  Kalman filter/3(a_rel) -> a_rel/1
  initial_value/1 -> Kalman filter/4(initial_value)
  cut_in_flg/1 -> Kalman filter/1(cut_in_flg)

== system acc/acceleration_apr1 ==
  acc_b : Inport
  Abs : Abs
  Constant1 : Constant  Value=0
  Switch : Switch  Criteria=u2 > Threshold  Threshold=0.01
  acc_a : Outport  VectorParamsAs1DForOutWhenUnconnected=off
  wires:
  Switch/1 -> acc_a/1
  acc_b/1 -> Abs/1, Switch/1
  Constant1/1 -> Switch/3
  Abs/1 -> Switch/2

== system acc/acceleration_apr4 ==
  acc_b : Inport
  Abs : Abs
  Constant1 : Constant  Value=0
  Switch : Switch  Criteria=u2 > Threshold  Threshold=0.01
  acc_a : Outport  VectorParamsAs1DForOutWhenUnconnected=off
  wires:
  Abs/1 -> Switch/2
  Constant1/1 -> Switch/3
  acc_b/1 -> Switch/1, Abs/1
  Switch/1 -> acc_a/1

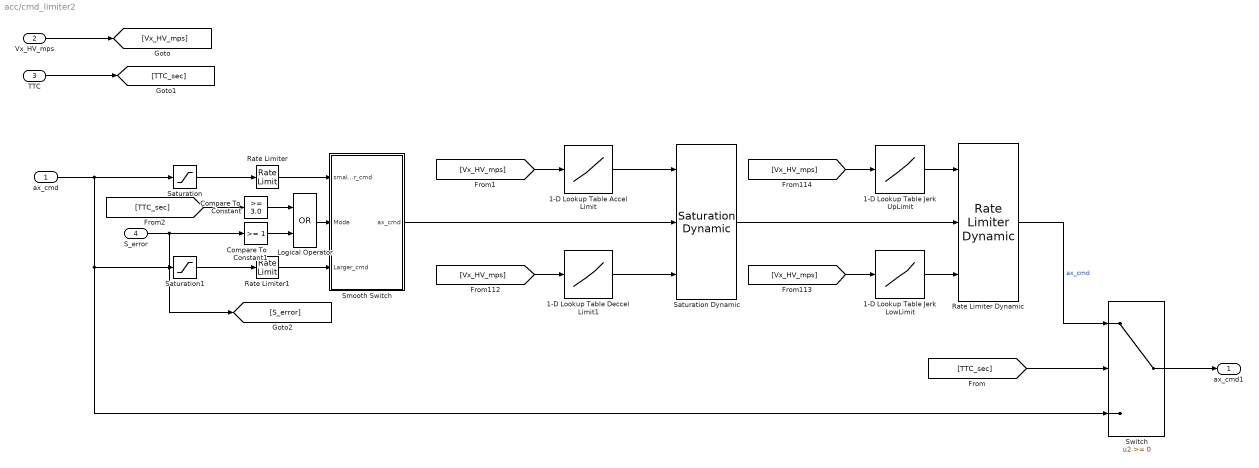
== system acc/cmd_limiter2 ==
  ax_cmd : Inport
  Vx_HV_mps : Inport  Port=2
  TTC : Inport  Port=3
  S_error : Inport  Port=4
  1-D Lookup Table Accel Limit : Lookup_n-D  NumberOfTableDimensions=1  BreakpointsForDimension1=[0,5,20,30]  Table=[4,4,2,2]  InternalRulePriority=Speed  RndMeth=Simplest  InputSameDT=on
  1-D Lookup Table Deccel Limit1 : Lookup_n-D  NumberOfTableDimensions=1  BreakpointsForDimension1=[0,5,20,30]  Table=[-5,-5,-2.5,-2.5]  InternalRulePriority=Speed  RndMeth=Simplest  InputSameDT=on
  1-D Lookup Table Jerk LowLimit : Lookup_n-D  NumberOfTableDimensions=1  BreakpointsForDimension1=[0,5,20,30]  Table=[-5,-5,-2.5,-2.5]  InternalRulePriority=Speed  RndMeth=Simplest  InputSameDT=on
  1-D Lookup Table Jerk UpLimit : Lookup_n-D  NumberOfTableDimensions=1  BreakpointsForDimension1=[0,5,20,30]  Table=[5,5,2.5,2.5]  InternalRulePriority=Speed  RndMeth=Simplest  InputSameDT=on
  Compare To Constant : simulink/Logic and Bit Operations/Compare To Constant  relop=>=  const=3.0  OutDataTypeStr=boolean
  Compare To Constant1 : simulink/Logic and Bit Operations/Compare To Constant  relop=>=  const=1  OutDataTypeStr=boolean
  Logical Operator : Logic  Operator=OR  AllPortsSameDT=off  OutDataTypeStr=boolean
  Rate Limiter : RateLimiter  RisingSlewLimit=2.5  FallingSlewLimit=-2.5  SampleTimeMode=inherited
  Rate Limiter Dynamic : simulink/Discontinuities/Rate Limiter Dynamic
  Rate Limiter1 : RateLimiter  RisingSlewLimit=2.5  FallingSlewLimit=-2.5  SampleTimeMode=inherited
  Saturation : Saturate  UpperLimit=2  LowerLimit=-2
  Saturation Dynamic : simulink/Discontinuities/Saturation Dynamic  OutMin=[]  OutMax=[]  OutDataTypeStr=Inherit: Same as second input  OutDataType=fixdt(1, 16)  OutScaling=2^-10  DoSatur=off
  Saturation1 : Saturate  UpperLimit=2  LowerLimit=-2
  Smooth Switch : Subsystem
  Switch : Switch
  ax_cmd1 : Outport
  wires:
  1-D Lookup Table Accel Limit/1 -> Saturation Dynamic/1
  [Vx_HV_mps] -> 1-D Lookup Table Jerk UpLimit/1
  1-D Lookup Table Jerk UpLimit/1 -> Rate Limiter Dynamic/1
  [Vx_HV_mps] -> 1-D Lookup Table Deccel Limit1/1
  [Vx_HV_mps] -> 1-D Lookup Table Jerk LowLimit/1
  1-D Lookup Table Deccel Limit1/1 -> Saturation Dynamic/3
  1-D Lookup Table Jerk LowLimit/1 -> Rate Limiter Dynamic/3
  Vx_HV_mps/1 -> [Vx_HV_mps]
  Saturation Dynamic/1 -> Rate Limiter Dynamic/2
  Rate Limiter Dynamic/1 -> Switch/1  "ax_cmd"
  [TTC_sec] -> Switch/2
  TTC/1 -> [TTC_sec]
  Smooth Switch/1(ax_cmd) -> Saturation Dynamic/2
  [Vx_HV_mps] -> 1-D Lookup Table Accel Limit/1
  Saturation/1 -> Rate Limiter/1
  ax_cmd/1 -> Saturation/1, Switch/3, Saturation1/1
  [TTC_sec] -> Compare To Constant/1
  Compare To Constant/1 -> Logical Operator/1
  Logical Operator/1 -> Smooth Switch/2(Mode)
  Compare To Constant1/1 -> Logical Operator/2
  S_error/1 -> [S_error], Compare To Constant1/1
  Rate Limiter/1 -> Smooth Switch/1(smaller_cmd)
  Rate Limiter1/1 -> Smooth Switch/3(Larger_cmd)
  Saturation1/1 -> Rate Limiter1/1
  Switch/1 -> ax_cmd1/1

== system acc/cmd_limiter3 ==
  ax_cmd : Inport
  Vx_HV_mps : Inport  Port=2
  TTC : Inport  Port=3
  1-D Lookup Table Accel Limit : Lookup_n-D  NumberOfTableDimensions=1  BreakpointsForDimension1=[0,5,20,30]  Table=[4,4,2,2]  InternalRulePriority=Speed  RndMeth=Simplest  InputSameDT=on
  1-D Lookup Table Deccel Limit1 : Lookup_n-D  NumberOfTableDimensions=1  BreakpointsForDimension1=[0,5,20,30]  Table=[-5,-5,-2.5,-2.5]  InternalRulePriority=Speed  RndMeth=Simplest  InputSameDT=on
  1-D Lookup Table Jerk LowLimit : Lookup_n-D  NumberOfTableDimensions=1  BreakpointsForDimension1=[0,5,20,30]  Table=[-5,-5,-2.5,-2.5]  InternalRulePriority=Speed  RndMeth=Simplest  InputSameDT=on
  1-D Lookup Table Jerk UpLimit : Lookup_n-D  NumberOfTableDimensions=1  BreakpointsForDimension1=[0,5,20,30]  Table=[5,5,2.5,2.5]  InternalRulePriority=Speed  RndMeth=Simplest  InputSameDT=on
  Compare To Constant : simulink/Logic and Bit Operations/Compare To Constant  relop=>=  const=3.0  OutDataTypeStr=boolean
  Rate Limiter : RateLimiter  RisingSlewLimit=2.5  FallingSlewLimit=-2.5  SampleTimeMode=inherited
  Rate Limiter Dynamic : simulink/Discontinuities/Rate Limiter Dynamic
  Saturation : Saturate  UpperLimit=2  LowerLimit=-2
  Saturation Dynamic : simulink/Discontinuities/Saturation Dynamic  OutMin=[]  OutMax=[]  OutDataTypeStr=Inherit: Same as second input  OutDataType=fixdt(1, 16)  OutScaling=2^-10  DoSatur=off
  Smooth Switch : Subsystem
  Switch : Switch
  Switch1 : Switch  Threshold=3
  ax_cmd1 : Outport
  wires:
  Compare To Constant/1 -> Smooth Switch/2(Mode)
  [TTC_sec] -> Compare To Constant/1
  Rate Limiter/1 -> Switch1/1, Smooth Switch/1(smaller_cmd)
  Saturation/1 -> Rate Limiter/1
  [Vx_HV_mps] -> 1-D Lookup Table Accel Limit/1
  Smooth Switch/1(ax_cmd) -> Saturation Dynamic/2
  TTC/1 -> [TTC_sec], Switch1/2
  Switch/1 -> ax_cmd1/1
  [TTC_sec] -> Switch/2
  Rate Limiter Dynamic/1 -> Switch/1  "ax_cmd"
  ax_cmd/1 -> Switch/3, Switch1/3, Smooth Switch/3(Larger_cmd), Saturation/1
  Saturation Dynamic/1 -> Rate Limiter Dynamic/2
  Vx_HV_mps/1 -> [Vx_HV_mps]
  1-D Lookup Table Jerk LowLimit/1 -> Rate Limiter Dynamic/3
  1-D Lookup Table Deccel Limit1/1 -> Saturation Dynamic/3
  [Vx_HV_mps] -> 1-D Lookup Table Jerk LowLimit/1
  [Vx_HV_mps] -> 1-D Lookup Table Deccel Limit1/1
  1-D Lookup Table Jerk UpLimit/1 -> Rate Limiter Dynamic/1
  [Vx_HV_mps] -> 1-D Lookup Table Jerk UpLimit/1
  1-D Lookup Table Accel Limit/1 -> Saturation Dynamic/1

== system acc/divide ==
  dividend : Inport
  divisor : Inport  Port=2
  default_value : Inport  Port=3
  Divide : Product  Inputs=*/
  Interval Test : simulink/Logic and Bit Operations/Interval Test  IntervalClosedRight=on  uplimit=5  IntervalClosedLeft=on  lowlimit=-1  OutDataTypeStr=boolean
  Logical Operator : Logic  Operator=NOT  Inputs=1  AllPortsSameDT=off  OutDataTypeStr=boolean
  Scope : Scope
  Switch : Switch  Criteria=u2 ~= 0  Threshold=0.5
  quotient : Outport
  wires:
  Logical Operator/1 -> Switch/2
  default_value/1 -> Switch/3  "default_value"
  Interval Test/1 -> Scope/1, Logical Operator/1
  Switch/1 -> quotient/1
  Divide/1 -> Switch/1
  divisor/1 -> Interval Test/1, Divide/2  "divisor"
  dividend/1 -> Divide/1  "dividend"

== system acc/divide1 ==
  dividend : Inport
  divisor : Inport  Port=2
  default_value : Inport  Port=3
  Divide : Product  Inputs=*/
  Interval Test : simulink/Logic and Bit Operations/Interval Test  IntervalClosedRight=on  uplimit=1  IntervalClosedLeft=on  lowlimit=-1  OutDataTypeStr=boolean
  Logical Operator : Logic  Operator=NOT  Inputs=1  AllPortsSameDT=off  OutDataTypeStr=boolean
  Scope : Scope
  Switch : Switch  Criteria=u2 ~= 0  Threshold=0.5
  quotient : Outport
  wires:
  Logical Operator/1 -> Switch/2
  default_value/1 -> Switch/3  "default_value"
  Interval Test/1 -> Scope/1, Logical Operator/1
  Switch/1 -> quotient/1
  Divide/1 -> Switch/1
  divisor/1 -> Interval Test/1, Divide/2  "divisor"
  dividend/1 -> Divide/1  "dividend"

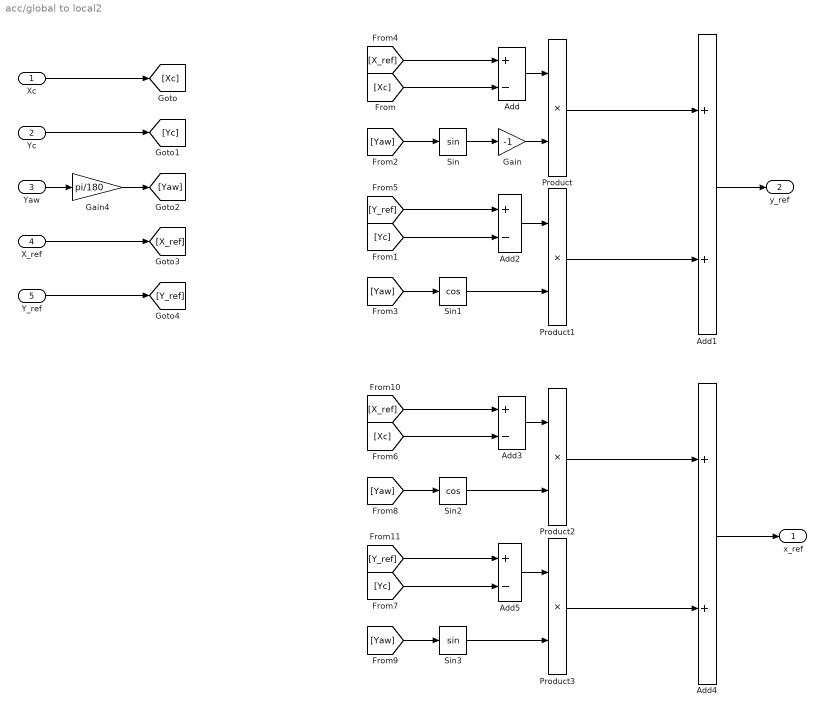
== system acc/global to local2 ==
  Xc : Inport
  Yc : Inport  Port=2
  Yaw : Inport  Port=3
  X_ref : Inport  Port=4
  Y_ref : Inport  Port=5
  Add{,2..3,5} (4 alike) : Sum  Inputs=+-
  Add1 : Sum
  Add4 : Sum
  Gain : Gain  Gain=-1
  Gain4 : Gain  Gain=pi/180
  Product{,1..3} (4 alike) : Product
  Sin : Trigonometry
  Sin1 : Trigonometry  Operator=cos
  Sin2 : Trigonometry  Operator=cos
  Sin3 : Trigonometry
  x_ref : Outport
  y_ref : Outport  Port=2
  wires:
  [X_ref] -> Add3/1
  [Y_ref] -> Add5/1
  Sin2/1 -> Product2/2
  Add3/1 -> Product2/1
  Product2/1 -> Add4/1
  Sin3/1 -> Product3/2
  Add5/1 -> Product3/1
  Product3/1 -> Add4/2
  Add4/1 -> x_ref/1
  [Yaw] -> Sin2/1
  [Yc] -> Add5/2
  [Xc] -> Add3/2
  [Yaw] -> Sin3/1
  Gain4/1 -> [Yaw]
  Y_ref/1 -> [Y_ref]
  X_ref/1 -> [X_ref]
  [Yaw] -> Sin1/1
  Yaw/1 -> Gain4/1
  Yc/1 -> [Yc]
  Xc/1 -> [Xc]
  [Xc] -> Add/2
  [Yc] -> Add2/2
  [Yaw] -> Sin/1
  Add1/1 -> y_ref/1
  Product1/1 -> Add1/2
  Add2/1 -> Product1/1
  Sin1/1 -> Product1/2
  Product/1 -> Add1/1
  Add/1 -> Product/1
  Gain/1 -> Product/2
  Sin/1 -> Gain/1
  [Y_ref] -> Add2/1
  [X_ref] -> Add/1

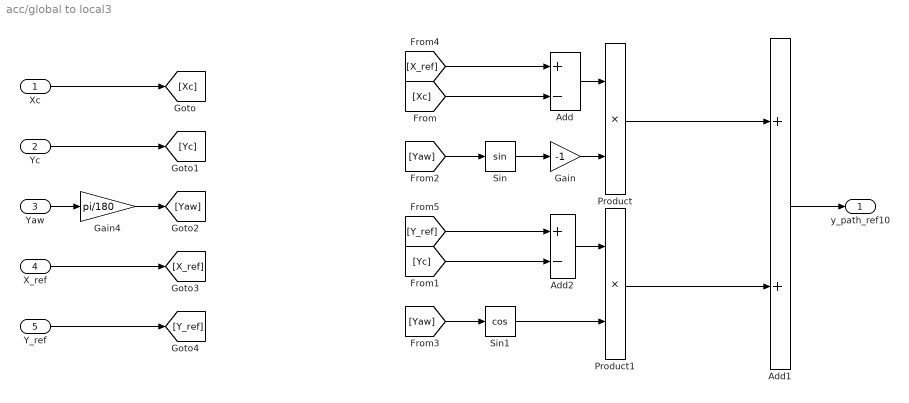
== system acc/global to local3 ==
  Xc : Inport
  Yc : Inport  Port=2
  Yaw : Inport  Port=3
  X_ref : Inport  Port=4
  Y_ref : Inport  Port=5
  Add : Sum  Inputs=+-
  Add1 : Sum
  Add2 : Sum  Inputs=+-
  Gain : Gain  Gain=-1
  Gain4 : Gain  Gain=pi/180
  Product : Product
  Product1 : Product
  Sin : Trigonometry
  Sin1 : Trigonometry  Operator=cos
  y_path_ref10 : Outport
  wires:
  Gain4/1 -> [Yaw]
  Y_ref/1 -> [Y_ref]
  X_ref/1 -> [X_ref]
  [Yaw] -> Sin1/1
  Yaw/1 -> Gain4/1
  Yc/1 -> [Yc]
  Xc/1 -> [Xc]
  [Xc] -> Add/2
  [Yc] -> Add2/2
  [Yaw] -> Sin/1
  Add1/1 -> y_path_ref10/1
  Product1/1 -> Add1/2
  Add2/1 -> Product1/1
  Sin1/1 -> Product1/2
  Product/1 -> Add1/1
  Add/1 -> Product/1
  Gain/1 -> Product/2
  Sin/1 -> Gain/1
  [Y_ref] -> Add2/1
  [X_ref] -> Add/1

== system acc/preview ==
  In1 : Inport
  In2 : Inport  Port=2
  Add9 : Sum
  Constant20 : Constant  Value=s_path
  Constant21 : Constant  Value=X_path
  Constant22 : Constant  Value=s_path
  Constant23 : Constant  Value=Y_path
  Constant49 : Constant  Value=[1:10]'
  Constant51 : Constant  Value=0.1
  Demux4 : Demux  Outputs=[1 9]
  Demux5 : Demux  Outputs=[1 9]
  Lookup Table Dynamic : simulink/Lookup Tables/Lookup Table Dynamic  LookUpMeth=Interpolation-Use End Values  OutDataType=fixdt('double')  OutScaling=[]  OutputDataTypeScalingMode=Specify via dialog  OutDataTypeStr=double  DoSatur=off
  Lookup Table Dynamic1 : simulink/Lookup Tables/Lookup Table Dynamic  LookUpMeth=Interpolation-Use End Values  OutDataType=fixdt('double')  OutScaling=[]  OutputDataTypeScalingMode=Specify via dialog  OutDataTypeStr=double  DoSatur=off
  Product1 : Product
  Product10 : Product
  Scope7 : Scope
  Terminator : Terminator
  Terminator1 : Terminator
  To Workspace27 : ToWorkspace  VariableName=X_ref  SampleTime=-1
  To Workspace28 : ToWorkspace  VariableName=Y_ref  SampleTime=-1
  X_ref : Outport
  Y_ref : Outport  Port=2
  wires:
  Constant23/1 -> Lookup Table Dynamic1/3
  Product10/1 -> Add9/2
  Product1/1 -> Product10/2
  Constant22/1 -> Lookup Table Dynamic1/2
  Constant20/1 -> Lookup Table Dynamic/2
  Constant21/1 -> Lookup Table Dynamic/3
  Lookup Table Dynamic1/1 -> Y_ref/1, Demux5/1
  Demux5/1 -> To Workspace28/1
  In1/1 -> Add9/1
  Lookup Table Dynamic/1 -> X_ref/1, Demux4/1
  In2/1 -> Product10/1
  Constant51/1 -> Product1/2
  Add9/1 -> Lookup Table Dynamic1/1, Scope7/1, Lookup Table Dynamic/1
  Constant49/1 -> Product1/1
  Demux4/1 -> To Workspace27/1
  Demux5/2 -> Terminator1/1
  Demux4/2 -> Terminator/1

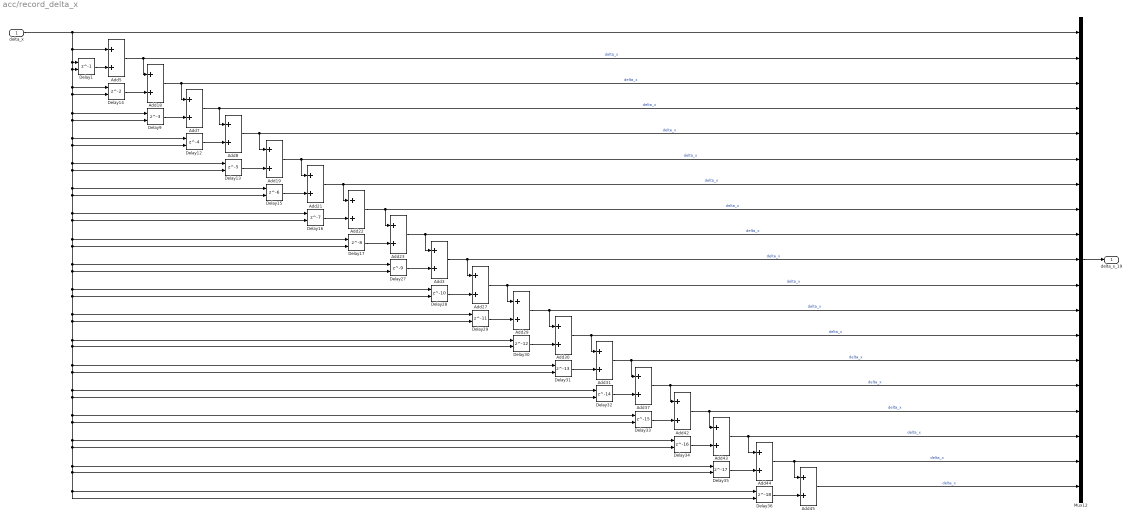
== system acc/record_delta_x ==
  delta_x : Inport
  Add{3,5,7..8,18..19,21..23,27,29..31,37,42..45} (18 alike) : Sum
  Delay1 : Delay  DelayLength=1  InitialConditionSource=Input port
      settings: InputPortMap=u0,p4
  Delay12 : Delay  DelayLength=4  InitialConditionSource=Input port
      settings: InputPortMap=u0,p4
  Delay13 : Delay  DelayLength=5  InitialConditionSource=Input port
      settings: InputPortMap=u0,p4
  Delay14 : Delay  InitialConditionSource=Input port
      settings: InputPortMap=u0,p4
  Delay15 : Delay  DelayLength=6  InitialConditionSource=Input port
      settings: InputPortMap=u0,p4
  Delay16 : Delay  DelayLength=7  InitialConditionSource=Input port
      settings: InputPortMap=u0,p4
  Delay17 : Delay  DelayLength=8  InitialConditionSource=Input port
      settings: InputPortMap=u0,p4
  Delay27 : Delay  DelayLength=9  InitialConditionSource=Input port
      settings: InputPortMap=u0,p4
  Delay28 : Delay  DelayLength=10  InitialConditionSource=Input port
      settings: InputPortMap=u0,p4
  Delay29 : Delay  DelayLength=11  InitialConditionSource=Input port
      settings: InputPortMap=u0,p4
  Delay30 : Delay  DelayLength=12  InitialConditionSource=Input port
      settings: InputPortMap=u0,p4
  Delay31 : Delay  DelayLength=13  InitialConditionSource=Input port
      settings: InputPortMap=u0,p4
  Delay32 : Delay  DelayLength=14  InitialConditionSource=Input port
      settings: InputPortMap=u0,p4
  Delay33 : Delay  DelayLength=15  InitialConditionSource=Input port
      settings: InputPortMap=u0,p4
  Delay34 : Delay  DelayLength=16  InitialConditionSource=Input port
      settings: InputPortMap=u0,p4
  Delay35 : Delay  DelayLength=17  InitialConditionSource=Input port
      settings: InputPortMap=u0,p4
  Delay36 : Delay  DelayLength=18  InitialConditionSource=Input port
      settings: InputPortMap=u0,p4
  Delay9 : Delay  DelayLength=3  InitialConditionSource=Input port
      settings: InputPortMap=u0,p4
  Mux12 : Mux  Inputs=19
  delta_x_19 : Outport
  wires:
  Add19/1 -> Mux12/6, Add21/1  "delta_x"
  Delay13/1 -> Add19/2
  Add44/1 -> Add45/1, Mux12/18  "delta_x"
  delta_x/1 -> Mux12/1, Delay14/2, Delay9/1, Delay15/1, Delay27/2, Delay28/1, Delay30/2, Delay31/1, Delay32/1, Delay33/1, Delay33/2, Delay34/1, Delay35/1, Delay36/1, Delay36/2, Delay35/2, Delay34/2, Delay32/2, Delay31/2, Delay30/1, Delay29/2, Delay29/1, Delay28/2, Delay27/1, Delay17/2, Delay17/1, Delay16/2, Delay16/1, Delay15/2, Delay13/2, Delay13/1, Delay12/2, Delay12/1, Delay9/2, Delay14/1, Delay1/2, Delay1/1, Add5/1
  Add29/1 -> Mux12/12, Add30/1  "delta_x"
  Add5/1 -> Mux12/2, Add18/1  "delta_x"
  Add18/1 -> Mux12/3, Add7/1  "delta_x"
  Delay29/1 -> Add29/2
  Delay1/1 -> Add5/2
  Add31/1 -> Mux12/14, Add37/1  "delta_x"
  Delay33/1 -> Add42/2
  Add23/1 -> Mux12/9, Add3/1  "delta_x"
  Delay9/1 -> Add7/2
  Add42/1 -> Add43/1, Mux12/16  "delta_x"
  Mux12/1 -> delta_x_19/1
  Delay14/1 -> Add18/2
  Add21/1 -> Mux12/7, Add22/1  "delta_x"
  Add30/1 -> Mux12/13, Add31/1  "delta_x"
  Delay34/1 -> Add43/2
  Delay17/1 -> Add23/2
  Delay27/1 -> Add3/2
  Add45/1 -> Mux12/19  "delta_x"
  Delay31/1 -> Add31/2
  Add43/1 -> Add44/1, Mux12/17  "delta_x"
  Delay15/1 -> Add21/2
  Add8/1 -> Mux12/5, Add19/1  "delta_x"
  Delay32/1 -> Add37/2
  Delay35/1 -> Add44/2
  Delay36/1 -> Add45/2
  Add27/1 -> Mux12/11, Add29/1  "delta_x"
  Add3/1 -> Mux12/10, Add27/1  "delta_x"
  Delay28/1 -> Add27/2
  Delay16/1 -> Add22/2
  Add22/1 -> Mux12/8, Add23/1  "delta_x"
  Delay30/1 -> Add30/2
  Add37/1 -> Mux12/15, Add42/1  "delta_x"
  Delay12/1 -> Add8/2
  Add7/1 -> Mux12/4, Add8/1  "delta_x"

== system acc/record_delta_yaw ==
  delta_yaw : Inport
  Add78 : Sum  Inputs=+-
  Delay68 : Delay  DelayLength=1  InitialConditionSource=Input port
      settings: InputPortMap=u0,p4
  Delay69 : Delay  InitialConditionSource=Input port
      settings: InputPortMap=u0,p4
  Delay70 : Delay  DelayLength=3  InitialConditionSource=Input port
      settings: InputPortMap=u0,p4
  Delay71 : Delay  DelayLength=4  InitialConditionSource=Input port
      settings: InputPortMap=u0,p4
  Delay72 : Delay  DelayLength=5  InitialConditionSource=Input port
      settings: InputPortMap=u0,p4
  Delay73 : Delay  DelayLength=6  InitialConditionSource=Input port
      settings: InputPortMap=u0,p4
  Delay74 : Delay  DelayLength=7  InitialConditionSource=Input port
      settings: InputPortMap=u0,p4
  Delay75 : Delay  DelayLength=8  InitialConditionSource=Input port
      settings: InputPortMap=u0,p4
  Delay76 : Delay  DelayLength=9  InitialConditionSource=Input port
      settings: InputPortMap=u0,p4
  Delay77 : Delay  DelayLength=10  InitialConditionSource=Input port
      settings: InputPortMap=u0,p4
  Delay78 : Delay  DelayLength=11  InitialConditionSource=Input port
      settings: InputPortMap=u0,p4
  Delay79 : Delay  DelayLength=12  InitialConditionSource=Input port
      settings: InputPortMap=u0,p4
  Delay80 : Delay  DelayLength=13  InitialConditionSource=Input port
      settings: InputPortMap=u0,p4
  Delay81 : Delay  DelayLength=14  InitialConditionSource=Input port
      settings: InputPortMap=u0,p4
  Delay82 : Delay  DelayLength=15  InitialConditionSource=Input port
      settings: InputPortMap=u0,p4
  Delay83 : Delay  DelayLength=16  InitialConditionSource=Input port
      settings: InputPortMap=u0,p4
  Delay84 : Delay  DelayLength=17  InitialConditionSource=Input port
      settings: InputPortMap=u0,p4
  Delay85 : Delay  DelayLength=18  InitialConditionSource=Input port
      settings: InputPortMap=u0,p4
  Delay86 : Delay  DelayLength=19  InitialConditionSource=Input port
      settings: InputPortMap=u0,p4
  Mux18 : Mux  Inputs=19
  delta_yaw_19 : Outport
  wires:
  Delay84/1 -> Mux18/17
  Delay72/1 -> Mux18/5
  Delay73/1 -> Mux18/6
  Delay78/1 -> Mux18/11
  Delay71/1 -> Mux18/4
  Delay68/1 -> Mux18/1
  Delay76/1 -> Mux18/9
  delta_yaw/1 -> Delay68/1, Delay68/2, Delay86/2, Delay86/1, Delay85/2, Delay85/1, Delay84/2, Delay84/1, Delay83/2, Delay83/1, Delay82/2, Delay82/1, Delay81/2, Delay81/1, Delay80/2, Delay80/1, Delay79/2, Delay79/1, Delay78/2, Delay78/1, Delay77/2, Delay77/1, Delay76/2, Delay76/1, Delay75/2, Delay75/1, Delay74/2, Delay74/1, Delay73/2, Delay73/1, Delay72/2, Delay72/1, Delay71/2, Delay71/1, Delay70/2, Delay70/1, Delay69/2, Delay69/1, Add78/1
  Delay81/1 -> Mux18/14
  Delay75/1 -> Mux18/8
  Delay80/1 -> Mux18/13
  Delay86/1 -> Mux18/19
  Delay82/1 -> Mux18/15
  Delay69/1 -> Mux18/2
  Delay70/1 -> Mux18/3
  Delay74/1 -> Mux18/7
  Mux18/1 -> Add78/2
  Delay77/1 -> Mux18/10
  Add78/1 -> delta_yaw_19/1
  Delay85/1 -> Mux18/18
  Delay79/1 -> Mux18/12
  Delay83/1 -> Mux18/16
